simulink model "Trayectorias_T8_SML"  (R2021a)
settings: Solver=VariableStepAuto  StartTime=0.0  StopTime=30  RelTol=1e-3
settings Model: Creator=LAFB2000  LastModifiedBy=LAFB2000

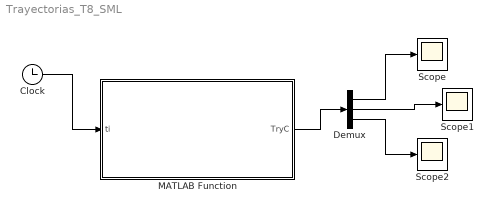
== system Trayectorias_T8_SML ==
  Clock : Clock
  Demux : Demux  Outputs=3
  MATLAB Function : MATLAB Function  TreatAsAtomicUnit=on
  Scope : Scope
  Scope1 : Scope
  Scope2 : Scope
  wires:
  Clock/1 -> MATLAB Function/1(ti)
  Demux/1 -> Scope/1
  Demux/2 -> Scope1/1
  Demux/3 -> Scope2/1
  MATLAB Function/1(TryC) -> Demux/1

== matlab function Trayectorias_T8_SML/MATLAB Function ==
  data: ti input; TryC output
function TryC = TRAYECTORIA_CARTESIANA(ti)
%%%%%%%%%%%%%%%%Primer tramo de trayectoria%%%%%%%%%%
if (0<=ti)&&(ti<10)

ti=0;
tf=10;

xi=0.0491;    %%%%%%HOME EN X%%%%%%%
xf=-0.257;

yi=0.238;            %%%%%%HOME EN Y%%%%%%%
yf=0.005;

zi=0.20;%%d1-h+0.19  %%%%%%HOME EN z%%%%%%%
zf=-0.150;

   
else
   
%%%%%%%%%%%%%%%%Segundo tramo de trayectoria%%%%%%%%%%  

             if (10<=ti)&&(ti<=30)

                              ti=10;
                              tf=30;

                              xi=-0.257;
                              xf=-0.10;

                              yi=0.005;
                              yf=0.1;

                              zi=-0.150;
                              zf=-0.130;
                             
             end
             
end
   
   
%%%%%%%%%%%%%%%%Coeficientes de los polinomios%%%%%%%%%%                              
                             
a5x=6*(xf-xi)/((tf-ti)^5);
a4x=-15*(xf-xi)/((tf-ti)^4);
a3x=10*(xf-xi)/((tf-ti)^3);
a2x=0;
a1x=0;
a0x=xi;

a5y=6*(yf-yi)/((tf-ti)^5);
a4y=-15*(yf-yi)/((tf-ti)^4);
a3y=10*(yf-yi)/((tf-ti)^3);
a2y=0;
a1y=0;
a0y=yi;

a5z=6*(zf-zi)/((tf-ti)^5);
a4z=-15*(zf-zi)/((tf-ti)^4);
a3z=10*(zf-zi)/((tf-ti)^3);
a2z=0;
a1z=0;
a0z=zf;

    if ti < 30
 
       
%%%%%%%%Posiciones deseadas%%%%%%%%%%%


   Xd=a0x+a1x*ti+a2x*ti^2+a3x*ti^3+a4x*ti^4+a5x*ti^5;
   Yd=a0y+a1y*ti+a2y*ti^2+a3y*ti^3+a4y*ti^4+a5y*ti^5;
   Zd=a0z+a1z*ti+a2z*ti^2+a3z*ti^3+a4z*ti^4+a5z*ti^5;
   
    else
     
         Xd=0.257;
         Yd=0.005;
         Zd=0.035;
     
    end
   
   
A1=poly(Xd);
Yd=poly(2);
poly(3)=Zd;
